simulink model "PID_Discreto"  (R2021a)
settings: Solver=FixedStepAuto  StartTime=0.0  StopTime=300  FixedStep=Ts  RelTol=1e-3
values from neighbouring files (symbols this model uses):
  td = Tu/8    [PID_Ku.m]
  ti = Tu/2    [PID_Ku.m]
  Ts = 1    [Real_Esta_Disc_Ref.m]    (also in untitled5.m = 0.1)
undefined symbols (not defined in the file or in its folder): kp, q0, q1, q2
libraries: pid_lib x1
settings Model: Creator=Sergio  LastModifiedBy=Sergio

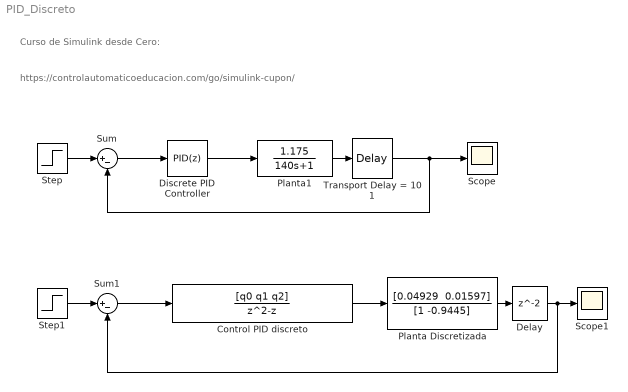
== system PID_Discreto ==
  note: Curso de Simulink desde Cero:
  note: https://controlautomaticoeducacion.com/go/simulink-cupon/
  Control PID discreto : DiscreteTransferFcn  Numerator=[q0 q1 q2]  Denominator=[1 -1 0]
  Delay : Delay  SampleTime=Ts
  Discrete PID Controller : pid_lib/PID Controller  Controller=PID  Form=Ideal  TimeDomain=Discrete-time  UseExternalTs=off  SampleTime=Ts  IntegratorMethod=Trapezoidal  FilterMethod=Trapezoidal  ControllerParametersSource=internal  P=kp  I=1/ti  D=td  UseFilter=off  N=100  TunerSelectOption=Transfer Function Based (PID Tuner App)  InitialConditionSource=internal  InitialConditionForIntegrator=0  InitialConditionForFilter=0  DifferentiatorICPrevScaledInput=0  ExternalReset=none  TrackingMode=off  Kt=1  LimitOutput=off  SatLimitsSource=internal  UpperSaturationLimit=inf  LowerSaturationLimit=-inf  LinearizeAsGain=off  AntiWindupMode=none  Kb=1  POutMin=[]  POutMax=[]  IOutMin=[]  IOutMax=[]  DOutMin=[]  DOutMax=[]  NOutMin=[]  NOutMax=[]  SumOutMin=[]  SumOutMax=[]  SaturationOutMin=[]  SaturationOutMax=[]  PParamMin=[]  PParamMax=[]  IParamMin=[]  IParamMax=[]  DParamMin=[]  DParamMax=[]  NParamMin=[]  NParamMax=[]  KbParamMin=[]  KbParamMax=[]  KtParamMin=[]  KtParamMax=[]  KbOutMin=[]  KbOutMax=[]  KtOutMin=[]  KtOutMax=[]  IntegratorOutMin=[]  IntegratorOutMax=[]  FilterOutMin=[]  FilterOutMax=[]  SumI1OutMin=[]  SumI1OutMax=[]  SumI2OutMin=[]  SumI2OutMax=[]  SumI3OutMin=[]  SumI3OutMax=[]  SumI4OutMin=[]  SumI4OutMax=[]  SumDOutMin=[]  SumDOutMax=[]  DifferentiatorOutMin=[]  DifferentiatorOutMax=[]  FilterDiffOutCoefMin=[]  FilterDiffOutCoefMax=[]  ReciprocalOutMin=[]  ReciprocalOutMax=[]  SumDenOutMin=[]  SumDenOutMax=[]  SumNumOutMin=[]  SumNumOutMax=[]  DivideOutMin=[]  DivideOutMax=[]  UdiffTsProdOutMin=[]  UdiffTsProdOutMax=[]  NTsProdOutMin=[]  NTsProdOutMax=[]  UintegralTsProdOutMin=[]  UintegralTsProdOutMax=[]  UngainTsProdOutMin=[]  UngainTsProdOutMax=[]  IntegratorContinuousStateAttributes=''  IntegratorStateMustResolveToSignalObject=off  IntegratorRTWStateStorageClass=Auto  FilterContinuousStateAttributes=''  FilterStateMustResolveToSignalObject=off  FilterRTWStateStorageClass=Auto  ParallelPVariant=Passthrough  IdealPVariant=InternalParameters  IVariant=InternalParameters  DVariant=InternalParameters  IntegratorVariant=Discrete  SatVariant=Disabled  AWVariant=Passthrough  PCopyVariant=Disabled  TRVariant=Disabled  FdbkBlocksVariant=Forward  IdealPFdbkVariant=Disabled  SatFdbkVariant=Disabled  DerivativeFilterVariant=Differentiator  NVariant=Passthrough  NCopyVariant=Disabled_SignalSpec  FilterICVariant=InternalICsDifferentiator  IntegratorICVariant=InternalICs  ExternalResetVariant=Disabled  TRSumVariant=Passthrough  SumFdbkVariant=Disabled  SumVariant=Sum_PID  TsampFilterVariant=InternalTs  TsampNgainVariant=Passthrough  TsampIntegralVariant=Passthrough  ExternalSaturationOutDataTypeStr=Inherit: Same as second input
  Planta Discretizada : DiscreteFilter  Numerator="[0.04929  0.01597]"  Denominator=[1 -0.9445]  SampleTime=Ts
  Planta1 : TransferFcn  Numerator=[1.175]  Denominator=[140 1]
  Scope : Scope
  Scope1 : Scope
  Step : Step  Time=0  SampleTime=Ts
  Step1 : Step  Time=0  SampleTime=Ts
  Sum : Sum  Inputs=|+-
  Sum1 : Sum  Inputs=|+-
  Transport Delay = 10 1 : TransportDelay  DelayTime=10
  wires:
  Discrete PID Controller/1 -> Planta1/1
  Step/1 -> Sum/1
  Sum/1 -> Discrete PID Controller/1
  Transport Delay = 10 1/1 -> Sum/2, Scope/1
  Delay/1 -> Scope1/1, Sum1/2
  Step1/1 -> Sum1/1
  Sum1/1 -> Control PID discreto/1
  Control PID discreto/1 -> Planta Discretizada/1
  Planta Discretizada/1 -> Delay/1
  Planta1/1 -> Transport Delay = 10 1/1
